simulink model "FM"  (R2016a)
settings: Solver=ode3  StartTime=0.0  StopTime=5  FixedStep=1/2000000  RelTol=1e-3
libraries: dsparch4 x1, dspvision x1
settings Model: Creator=camj3302  LastModifiedBy=camj3302
settings SolverCC: AutoInsertRateTranBlk=on

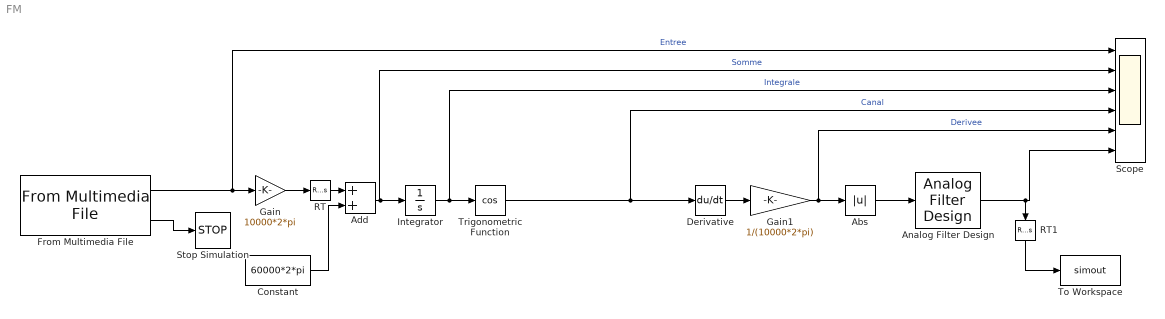
== system FM ==
  Abs : Abs
  Add : Sum
  Analog Filter Design : dsparch4/Analog Filter Design  method=Butterworth  filttype=Bandpass  N=10  Wlo=20*2*pi  Whi=20000*2*pi  Rp=2  Rs=40
  Constant : Constant  Value=60000*2*pi  SampleTime=1/2000000
  Derivative : Derivative
  From Multimedia File : dspvision/From Multimedia File  inputFilename=Q:\S6APP3\sons\son1.wav  loop=on  numPlays=1  outputStreams=Audio only  videoDataType=single  audioDataType=double  inheritSampleTime=on  userDefinedSampleTime=1/30  noAudioOutput=off  isIntensityVideo=off  fourcc=RGB  colorVideoFormat=Separate color signals  outputEOF=on  dataOrg=Column-major  audioFrameSize=1  computeAudioFrameSize=off  outSamplingMode=Sample based
  Gain : Gain  Gain=10000*2*pi
  Gain1 : Gain  Gain=1/(10000*2*pi)
  Integrator : Integrator
  RT : RateTransition  OutPortSampleTime=5e-07
  RT1 : RateTransition  OutPortSampleTime=1/40000
  Scope : Scope  NumInputPorts=6
  Stop Simulation : Stop
  To Workspace : ToWorkspace  VariableName=simout  SampleTime=-1
      settings: Save2DSignal=2-D array (concatenate along first dimension)
  Trigonometric Function : Trigonometry  Operator=cos
  wires:
  From Multimedia File/1 -> Scope/1, Gain/1  "Entree"
  Gain/1 -> RT/1
  Constant/1 -> Add/2
  Add/1 -> Scope/2, Integrator/1  "Somme"
  Integrator/1 -> Scope/3, Trigonometric Function/1  "Integrale"
  Trigonometric Function/1 -> Derivative/1, Scope/4  "Canal"
  Derivative/1 -> Gain1/1
  Gain1/1 -> Scope/5, Abs/1  "Derivee"
  Abs/1 -> Analog Filter Design/1
  Analog Filter Design/1 -> Scope/6, RT1/1
  From Multimedia File/2 -> Stop Simulation/1
  RT/1 -> Add/1
  RT1/1 -> To Workspace/1
